simulink model "aufgabe_2"  (R2020b)
settings: Solver=VariableStepAuto  StartTime=0.0  StopTime=10.0  RelTol=1e-3
settings Model: Creator=fb3cei  LastModifiedBy=fb3cei

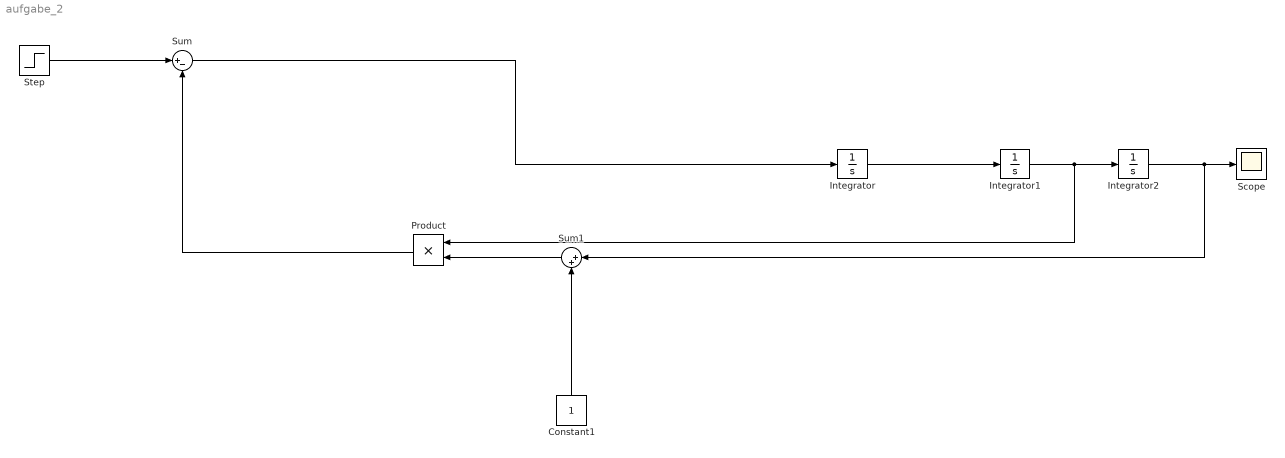
== system aufgabe_2 ==
  Constant1 : Constant
  Integrator : Integrator
  Integrator1 : Integrator
  Integrator2 : Integrator
  Product : Product
  Scope : Scope
  Step : Step  SampleTime=0
  Sum : Sum  Inputs=|+-
  Sum1 : Sum  Inputs=|++
  wires:
  Integrator2/1 -> Sum1/1, Scope/1
  Integrator/1 -> Integrator1/1
  Integrator1/1 -> Product/1, Integrator2/1
  Constant1/1 -> Sum1/2
  Sum1/1 -> Product/2
  Product/1 -> Sum/2
  Sum/1 -> Integrator/1
  Step/1 -> Sum/1
